simulink model "misura_PI_D"  (R2017a)
settings: Solver=VariableStepAuto  StartTime=0.0  StopTime=900  RelTol=1e-3
values from neighbouring files (symbols this model uses):
  N = 10    [metodo_grafico.m]
undefined symbols (not defined in the file or in its folder): kP, Td, Ti
libraries: cstblocks x1
settings Model: Creator=Enrico Donato  LastModifiedBy=Enrico Donato

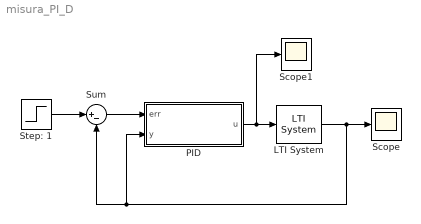
== system misura_PI_D ==
  LTI System : cstblocks/LTI System  sys=G  IC=[]
  "PID " : Subsystem
  Scope : Scope
  Scope1 : Scope
  Step: 1 : Step  Time=0  SampleTime=0
  Sum : Sum  Inputs=|+-
  wires:
  "PID "/1(u) -> LTI System/1, Scope1/1
  Sum/1 -> "PID "/1(err)
  Step: 1/1 -> Sum/1
  LTI System/1 -> "PID "/2("y "), Sum/2, Scope/1

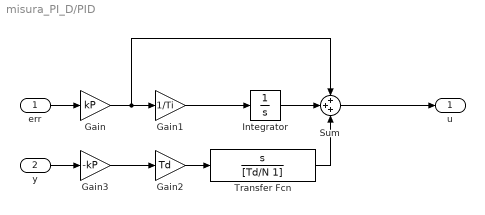
== system misura_PI_D/PID  ==
  err : Inport
  "y " : Inport  Port=2
  Gain : Gain  Gain=kP
  Gain1 : Gain  Gain=1/Ti
  Gain2 : Gain  Gain=Td
  Gain3 : Gain  Gain=-kP
  Integrator : Integrator
  Sum : Sum  Inputs=+++
  Transfer Fcn : TransferFcn  Numerator=[1 0]  Denominator=[Td/N 1]
  u : Outport
  wires:
  Sum/1 -> u/1
  err/1 -> Gain/1
  Gain1/1 -> Integrator/1
  Integrator/1 -> Sum/2
  Gain/1 -> Gain1/1, Sum/1
  Gain2/1 -> Transfer Fcn/1
  Gain3/1 -> Gain2/1
  "y "/1 -> Gain3/1
  Transfer Fcn/1 -> Sum/3
